simulink model "PID_Model"  (R2017a)
settings: Solver=VariableStepAuto  StartTime=0.0  StopTime=10.0  RelTol=1e-3
undefined symbols (not defined in the file or in its folder): G, Kd, Ki, Kp, N, N1, s
settings Model: Creator=Fouad  LastModifiedBy=Fouad

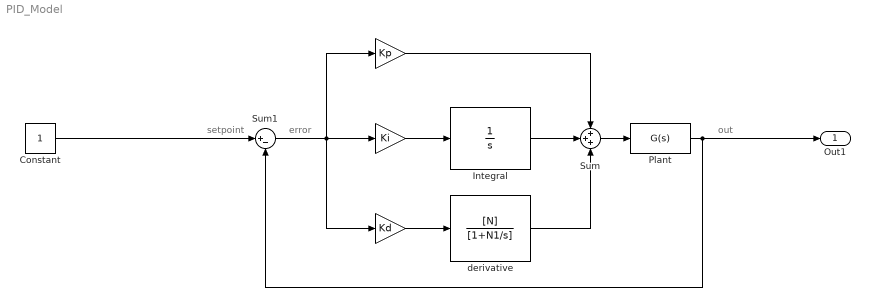
== system PID_Model ==
  note: setpoint
  note: out
  note: error
  " " : Gain  Gain=Kp
  " " : Gain  Gain=Ki
  " " : Gain  Gain=Kd
  Constant : Constant
  Integral : TransferFcn  Denominator=[1 0]
  Plant : Fcn  Expr=G(s)
  Sum : Sum  Inputs=+++
  Sum1 : Sum  Inputs=|+-
  derivative : TransferFcn  Numerator=[N]  Denominator=[1+N1/s]
  Out1 : Outport
  wires:
  " "/1 -> derivative/1
  " "/1 -> Integral/1
  derivative/1 -> Sum/3
  Integral/1 -> Sum/2
  Sum/1 -> Plant/1
  " "/1 -> Sum/1
  Sum1/1 -> " "/1, " "/1, " "/1
  Plant/1 -> Out1/1, Sum1/2
  Constant/1 -> Sum1/1
